simulink model "dioderect"  (R2016a)
settings: Solver=VariableStepAuto  StartTime=0.0  StopTime=10  RelTol=1e-3
libraries: powerlib x29
settings Model: Creator=hakan  LastModifiedBy=hakan

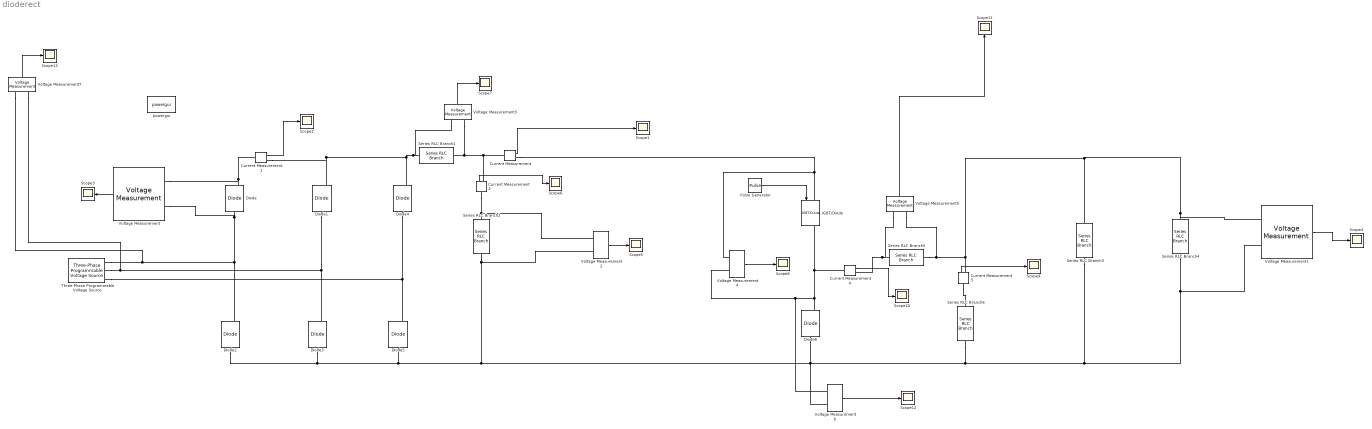
== system dioderect ==
  Current Measurement{,1..4} (5 alike) : powerlib/Measurements/Current Measurement  PhasorSimulation=off  OutputType=Complex  PSBequivalent=0
  Diode{,1..6} (7 alike) : powerlib/Power Electronics/Diode  Ron=0.001  Lon=0  Vf=0.8  IC=0  UseSnubber=off  Rs=500  Cs=250e-9  Measurements=on
  IGBT/Diode : powerlib/Power Electronics/IGBT//Diode  Ron=1e-3  Rs=1e5  Cs=inf  Measurements=on
  Pulse Generator : DiscretePulseGenerator  PulseType=Time based  Period=1/500  PulseWidth=80
  Scope{1..13} (13 alike) : Scope
  Series RLC Branch1 : powerlib/Elements/Series RLC Branch  LConnTagsString=__new0  RConnTagsString=__new0  BranchType=L  Resistance=30  Inductance=150e-3  SetiL0=off  InitialCurrent=0  Capacitance=1e-6  Setx0=off  InitialVoltage=0  Measurements=None
  Series RLC Branch2 : powerlib/Elements/Series RLC Branch  LConnTagsString=__new0  RConnTagsString=__new0  BranchType=C  Resistance=30  Inductance=13.3e-3  SetiL0=off  InitialCurrent=0  Capacitance=100e-6  Setx0=off  InitialVoltage=0  Measurements=None
  Series RLC Branch3 : powerlib/Elements/Series RLC Branch  LConnTagsString=__new0  RConnTagsString=__new0  BranchType=R  Resistance=17  Inductance=150e-3  SetiL0=off  InitialCurrent=0  Capacitance=1e-6  Setx0=off  InitialVoltage=0  Measurements=None
  Series RLC Branch4 : powerlib/Elements/Series RLC Branch  LConnTagsString=__new0  RConnTagsString=__new0  BranchType=R  Resistance=73  Inductance=150e-3  SetiL0=off  InitialCurrent=0  Capacitance=1e-6  Setx0=off  InitialVoltage=0  Measurements=None
  Series RLC Branch5 : powerlib/Elements/Series RLC Branch  LConnTagsString=__new0  RConnTagsString=__new0  BranchType=L  Resistance=30  Inductance=0.1  SetiL0=off  InitialCurrent=0  Capacitance=1e-6  Setx0=off  InitialVoltage=0  Measurements=None
  Series RLC Branch6 : powerlib/Elements/Series RLC Branch  LConnTagsString=__new0  RConnTagsString=__new0  BranchType=C  Resistance=30  Inductance=13.3e-3  SetiL0=off  InitialCurrent=0  Capacitance=150e-6  Setx0=off  InitialVoltage=0  Measurements=None
  Three-Phase Programmable Voltage Source : powerlib/Electrical Sources/Three-Phase Programmable Voltage Source  PositiveSequence="[120*sqrt(3)  0 50]"  VariationEntity=None  VariationType=Table of time-amplitude pairs  VariationTypeAlt=Step  VariationStep=0.5  VariationRate=10  VariationMagnitude=0.3  VariationFrequency=2  VariationTiming=[1 2]  VariationPhaseA=off  Amplitudes=[1 0.8 1.2 1.0]  TimeValues=[0 0.1 0.15 0.2]  HarmonicGeneration=off  HarmonicA=[3 0.2 -25 0]  HarmonicB=[2 0.15 35 2]  Timing="[0.05  3]"  BusType=swing  Pref=0  Qref=0  Qmin=-inf  Qmax=inf
  Voltage Measurement{,1..7} (8 alike) : powerlib/Measurements/Voltage Measurement  PhasorSimulation=off  OutputType=Complex  PSBequivalent=0
  powergui : powerlib/powergui  Priority=1  SimulationMode=Discrete  SolverType=Tustin/Backward Euler (TBE)  SampleTime=50e-6  frequency=60  SPID=off  DisableSnubberDevices=off  DisableRonSwitches=off  DisableVfSwitches=off  SwTol=0  DisplayEquations=off  Interpol=off  ExternalGateDelay=off  methode=off  Ts=10  FunctionMessages=off  echomessages=off  HookPort=off  EnableUseOfTLC=off  x0status=blocks  frequencyindice=50  Pbase=100e6  ErrMax=1e-4  Iterations=50  UnitsV=kV  UnitsW=MW  buscounter=0  RestoreLinks=warning  ResistiveCurrentMeasurement=off  Frange=[0:2:500]  Ylog=off  Xlog=on  ShowGrid=off  save=off  variable=ZData  structure=0  ZoomFFT=off  StartTime=0.0  cycles=1  DisplayStyle=1  fundamental=60  FreqAxis=off  MaxFrequency=1000  frequencyindicesteady=1  RmsSteady=1  display=off
  wires:
  Current Measurement/1 -> Scope1/1
  Current Measurement1/1 -> Scope2/1
  Voltage Measurement/1 -> Scope3/1
  Voltage Measurement1/1 -> Scope4/1
  Pulse Generator/1 -> IGBT/Diode/1
  Voltage Measurement2/1 -> Scope5/1
  Current Measurement2/1 -> Scope6/1
  Voltage Measurement3/1 -> Scope7/1
  Voltage Measurement4/1 -> Scope8/1
  Current Measurement3/1 -> Scope9/1
  Current Measurement4/1 -> Scope10/1
  Voltage Measurement5/1 -> Scope11/1
  Voltage Measurement6/1 -> Scope12/1
  Voltage Measurement7/1 -> Scope13/1
  connections:
  Diode/LConn1 -- Voltage Measurement7/LConn1 -- Three-Phase Programmable Voltage Source/RConn1 -- Diode2/RConn1 -- Voltage Measurement/LConn2
  Diode1/LConn1 -- Voltage Measurement7/LConn2 -- Three-Phase Programmable Voltage Source/RConn2 -- Diode3/RConn1
  Diode4/LConn1 -- Three-Phase Programmable Voltage Source/RConn3 -- Diode5/RConn1
  Series RLC Branch1/RConn1 -- Current Measurement1/RConn1 -- Diode1/RConn1 -- Diode4/RConn1 -- Voltage Measurement3/LConn1
  Series RLC Branch5/LConn1 -- Voltage Measurement5/LConn2 -- Series RLC Branch3/RConn1 -- Series RLC Branch4/RConn1 -- Voltage Measurement1/LConn1 -- Current Measurement3/RConn1
  Series RLC Branch2/LConn1 -- Current Measurement2/LConn1 -- Voltage Measurement2/LConn1
  Series RLC Branch2/RConn1 -- Voltage Measurement6/LConn2 -- Series RLC Branch6/RConn1 -- Voltage Measurement1/LConn2 -- Series RLC Branch4/LConn1 -- Series RLC Branch3/LConn1 -- Diode6/LConn1 -- Diode3/LConn1 -- Diode2/LConn1 -- Diode5/LConn1 -- Voltage Measurement2/LConn2
  Diode/RConn1 -- Current Measurement1/LConn1 -- Voltage Measurement/LConn1
  Current Measurement/RConn1 -- IGBT/Diode/LConn1 -- Voltage Measurement4/LConn1
  Series RLC Branch5/RConn1 -- Current Measurement4/RConn1 -- Voltage Measurement5/LConn1
  Current Measurement/LConn1 -- Current Measurement2/RConn1 -- Series RLC Branch1/LConn1 -- Voltage Measurement3/LConn2
  Current Measurement3/LConn1 -- Series RLC Branch6/LConn1
  Diode6/RConn1 -- Voltage Measurement6/LConn1 -- Voltage Measurement4/LConn2 -- IGBT/Diode/RConn1 -- Current Measurement4/LConn1
